simulink model "QAM"  (Simulink 10.3)
settings: Solver=VariableStepAuto  StartTime=0.0  StopTime=1000.0  RelTol=1e-3
undefined symbols (not defined in the file): j
libraries: dsp_blocks x7
settings Model: Creator=nathanalemayehu  LastModifiedBy=nathanalemayehu
settings SolverCC: AlgebraicLoopSolver=Auto
settings DataIOCC: SaveFormat=Dataset  SignalLoggingSaveFormat=Dataset  ReturnWorkspaceOutputs=on
settings OptimizationCC: ExpressionDepthLimit=128  LifeSpan=auto
settings DebuggingCC: UnderspecifiedInitializationDetection=Simplified  MergeDetectMultiDrivingBlocksExec=error  FcnCallInpInsideContextMsg=error  StateNameClashWarn=none  SFUnexpectedBacktrackingDiag=error  SFNoUnconditionalDefaultTransitionDiag=error  SFExecutionAtInitializationDiag=warning  SFMachineParentedDataDiag=error  ArithmeticOperatorsInVariantConditions=error
settings HardwareCC: ProdBitPerPointer=64  ProdBitPerSizeT=64  ProdBitPerPtrDiffT=64  ProdLargestAtomicFloat=Float  ProdIntDivRoundTo=Zero  ProdEndianess=LittleEndian  ProdWordSize=64  ProdHWDeviceType=Intel->x86-64 (Windows64)
settings ModelReferenceCC: PropagateSignalLabelsOutOfModel=on
settings SFSimCC: SimUseLocalCustomCode=on  CustomCodeUndefinedFunction=FilterOut
settings RTWCC: RTWUseLocalCustomCode=on
settings CodeAppCC: StateflowObjectComments=off
settings GRTTargetCC: TargetLangStandard=C99 (ISO)  CombineOutputUpdateFcns=on  GRTInterface=off
settings ConfigComp: CovMetricSettings=dwe  CovSaveCumulativeToWorkspaceVar=off  CovSaveSingleToWorkspaceVar=off  CovExternalEMLEnable=on

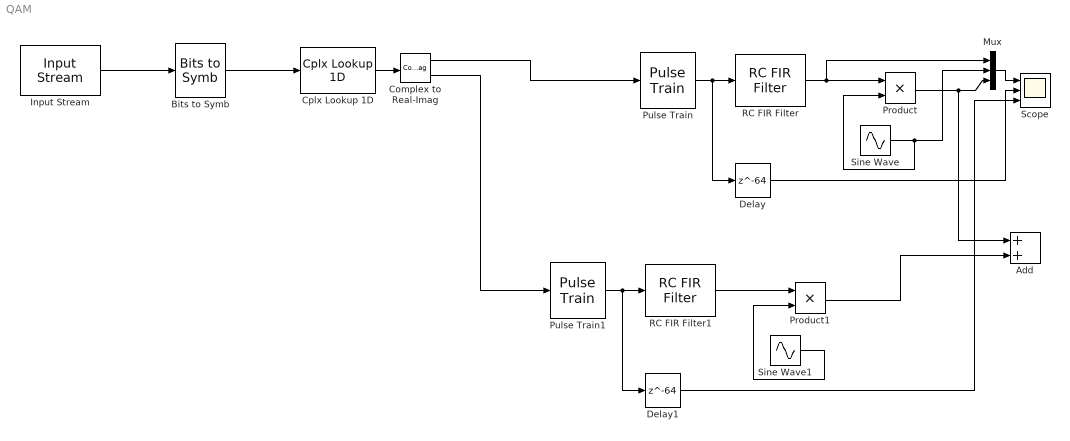
== system QAM ==
  Add : Sum
  Bits to Symb : dsp_blocks/Conversions/Bits to Symb
  Complex to Real-Imag : ComplexToRealImag
  Cplx Lookup 1D : dsp_blocks/Conversions/Cplx Lookup 1D  table=[1 j -1 -j]
  Delay : Delay  DelayLength=64
  Delay1 : Delay  DelayLength=64
  Input Stream : dsp_blocks/Sources//Sinks/Input Stream  period=50  width=2  fname=rand.mat
  Mux : Mux  Inputs=3
  Product : Product
  Product1 : Product
  Pulse Train : dsp_blocks/Conversions/Pulse Train  period=50
  Pulse Train1 : dsp_blocks/Conversions/Pulse Train  period=50
  RC FIR Filter : dsp_blocks/Filters/RC FIR Filter  period=50  beta=0.5  root=off  filt_len=128  win_type=on
  RC FIR Filter1 : dsp_blocks/Filters/RC FIR Filter  period=50  beta=0.5  root=off  filt_len=128  win_type=on
  Scope : Scope  NumInputPorts=3
  Sine Wave : Sin  Frequency=2*pi*0.1  Phase=pi/2  SampleTime=0
  Sine Wave1 : Sin  Frequency=2*pi*0.1  SampleTime=0
  wires:
  Product/1 -> Add/1, Mux/3
  RC FIR Filter1/1 -> Product1/1
  Bits to Symb/1 -> Cplx Lookup 1D/1
  Product1/1 -> Add/2
  Pulse Train/1 -> Delay/1, RC FIR Filter/1
  Sine Wave/1 -> Mux/2, Product/2
  RC FIR Filter/1 -> Mux/1, Product/1
  Delay/1 -> Scope/2
  Input Stream/1 -> Bits to Symb/1
  Cplx Lookup 1D/1 -> Complex to Real-Imag/1
  Sine Wave1/1 -> Product1/2
  Pulse Train1/1 -> Delay1/1, RC FIR Filter1/1
  Delay1/1 -> Scope/3
  Complex to Real-Imag/1 -> Pulse Train/1
  Mux/1 -> Scope/1
  Complex to Real-Imag/2 -> Pulse Train1/1
